simulink subsystem "SubSystemHubmagnetConveyor"  (R2020b)
settings: Solver=VariableStepAuto  StartTime=0.0  StopTime=10.0  RelTol=1e-3
settings Model: Creator=kaebi  LastModifiedBy=kaebi

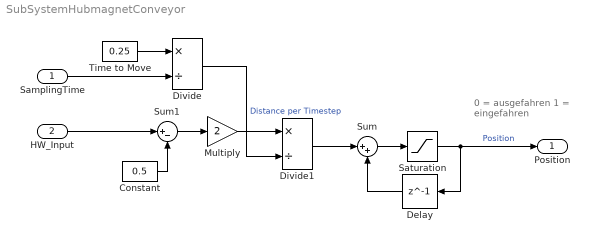
== system SubSystemHubmagnetConveyor ==
  note: 0 = ausgefahren
      | 1 = eingefahren
  SamplingTime : Inport
  HW_Input : Inport  Port=2
  Constant : Constant  Value=0.5
  Delay : Delay  DelayLength=1
  Divide : Product  Inputs=*/
  Divide1 : Product  Inputs=*/
  Multiply : Gain  Gain=2
  Saturation : Saturate  UpperLimit=1  LowerLimit=0
  Sum : Sum  Inputs=|++
  Sum1 : Sum  Inputs=|+-
  Time to Move : Constant  Value=0.25
  Position : Outport
  wires:
  Sum/1 -> Saturation/1
  Divide1/1 -> Sum/1
  Multiply/1 -> Divide1/1
  HW_Input/1 -> Sum1/1
  Saturation/1 -> Delay/1, Position/1  "Position"
  Sum1/1 -> Multiply/1
  Constant/1 -> Sum1/2
  Delay/1 -> Sum/2
  Divide/1 -> Divide1/2  "Distance per Timestep"
  SamplingTime/1 -> Divide/2
  Time to Move/1 -> Divide/1
